simulink model "simpleLogicStart"  (R2022b)
settings: Solver=VariableStepAuto  StartTime=0.0  StopTime=10.0  RelTol=1e-3  EnableMultiTasking=on
settings Model: Creator=jrivitus  LastModifiedBy=bensweet
settings SolverCC: AlgebraicLoopSolver=TrustRegion
settings DataIOCC: LimitDataPoints=on  SaveFormat=Array  ReturnWorkspaceOutputs=off
settings OptimizationCC: ExpressionDepthLimit=2147483647  InitFltsAndDblsToZero=on  LifeSpan=inf
settings DebuggingCC: UnconnectedInputMsg=warning  UnconnectedOutputMsg=warning  UnconnectedLineMsg=warning  PregeneratedLibrarySubsystemCodeDiagnostic=none  SFMachineParentedDataDiag=warning
settings HardwareCC: ProdBitPerPointer=32  ProdBitPerSizeT=32  ProdBitPerPtrDiffT=32  ProdLargestAtomicFloat=None  ProdIntDivRoundTo=Undefined  ProdEndianess=Unspecified  ProdWordSize=32  ProdHWDeviceType=32-bit Generic
settings ModelReferenceCC: EnableRefExpFcnMdlSchedulingChecks=on  PropagateSignalLabelsOutOfModel=off
settings SFSimCC: SimUseLocalCustomCode=off
settings RTWCC: RTWUseLocalCustomCode=off  DLArmComputeVersion=19.05
settings CodeAppCC: StateflowObjectComments=on
settings GRTTargetCC: TargetLangStandard=C89/C90 (ANSI)  CombineOutputUpdateFcns=off  GRTInterface=on
settings ConfigComp: CovMetricSettings=dw  CovSaveCumulativeToWorkspaceVar=on  CovSaveSingleToWorkspaceVar=on  CovExternalEMLEnable=off  CovSFcnEnable=off

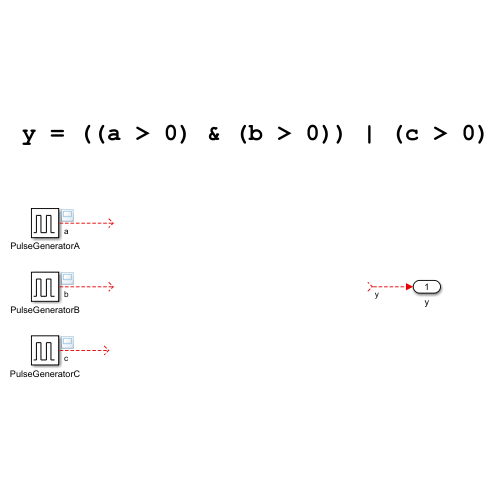
[thumbnail: Simulink's stored preview of the top-level diagram]
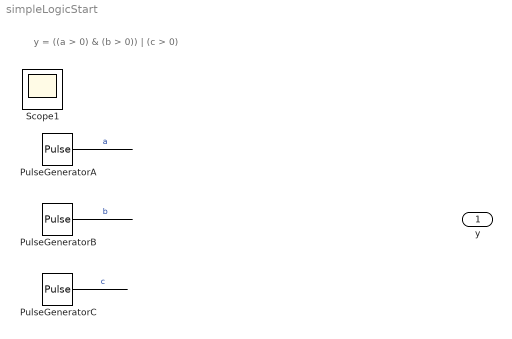
== system simpleLogicStart ==
  note: y = ((a > 0) & (b > 0)) | (c > 0)
  PulseGeneratorA : DiscretePulseGenerator  PulseType=Time based  Period=10  PulseWidth=20
  PulseGeneratorB : DiscretePulseGenerator  PulseType=Time based  Period=10  PulseWidth=20  PhaseDelay=1
  PulseGeneratorC : DiscretePulseGenerator  PulseType=Time based  Period=10  PulseWidth=20  PhaseDelay=7
  y : Outport  VectorParamsAs1DForOutWhenUnconnected=off
  Scope1 : Scope
  wires:
  ? -> y/1  "y"
  PulseGeneratorA/1 -> ?  "a"
  PulseGeneratorB/1 -> ?  "b"
  PulseGeneratorC/1 -> ?  "c"
